simulink model "Quaternions_Method_merge_main"  (R2021b)
settings: Solver=VariableStepAuto  StartTime=0.0  StopTime=Time  FixedStep=1e-1  RelTol=1e-13  AbsTol=1e-8
values from neighbouring files (symbols this model uses):
  a = 8.6251e06    (= 8625100)    [main_code.m]
  A_BN_0 = eye(3)    [main_code.m]
  A_rw = [1 0 0 1/sqrt(3);         0 1 0 1/sqrt(3) ... (first row only)    [main_code.m]
  A_rw_star = [5/6 -1/6 -1/6;              -1/6  5/6 -1/6 ... (first row only)    [main_code.m]
  c = 2.99792*10^8    (= 299792000)    [main_code.m]
  e = 0.1195    [main_code.m]
  i = 0.3815    [main_code.m]
  MB = [1; 0.3; 0.3; 0.3]    [main_code.m]
  mr = 1.2*1e-4    (= 0.00012)    [main_code.m]
  omega_0 = [w_0x; w_0y; w_0z]    [main_code.m]
  sig_b = sig_b^2    [main_code.m]
  sig_n = 0.15*pi/180/3600/sqrt(t_sample)    [main_code.m]
  SP = [3; 0.3; 1; 0.1]    [main_code.m]
  T = 2*pi / n    [main_code.m]
  t_sample = 1    [main_code.m]
undefined symbols (not defined in the file or in its folder): f_mag, H_0, magnitude, muP, p_acc, RD, RS_MB, RS_SP, theta0, w_E
libraries: matrix_library x14, vrlib x8, simulink x2, simulink_extras x1
(part 5 of 5)

== matlab function Quaternions_Method_merge_main/Attitude determination/MATLAB Function ==
  data: K input; V output; D output
function [V, D] = fcn(K)
[V,D] = eig(K);
end

== matlab function Quaternions_Method_merge_main/Enviroment/Magnetic torque /Magnetic torque in body frame/MATLAB Function ==
  data: R input; r_LVLH input; t input; teta input; B_N output
function B_N = fcn(R, r_LVLH, t, teta)

%% First thing is to define the vector containing all the polynimials up to the 4th order
P1 = 1;
P2 = teta;
P3 = ((3*teta^2)-1)/2;
P4 = ((5*teta^3)-(3*teta))/2;

% Computing the derivatives of the P polynomials
P1_der = 0;
P2_der = 1;
P3_der = 3*teta;
P4_der = ((15*teta^2)-3)/2;

r = norm(r_LVLH);
% Defining the order of the approximation k 
k = 4;

% Defining the matrices containing the coefficients needed to make the
% approximation model IGRF2000 (following the tables on the slide number 5 of the
% pack of slides number 8)
g = 1e9*[-29615 -1728 0 0 0; ...
                      -2267 3072 1672 0 0; ...
                     1341 -2290 1253 715 0; ...
                     935 787 251 -405 110]; %[T]
h = 1e9*[0 5186 0 0 0; ...
                     0 -2478 -458 0 0; ...
                     0 -227 296 -492 0; ...
                     0 272 -232 119 -304]; %[T]

% Computing the right ascension alpha, the declination delta, the longitude lon and the co-latitude phi
delta = asin(r_LVLH(3)/r); %[rad]
if(r_LVLH(2)/r > 0)
    alpha = acos((r_LVLH(1)/r)/cos(delta)); %[rad]
else 
    alpha = 2*pi -  acos((r_LVLH(1)/r)/cos(delta)); %[rad]
end
lat = -delta; %[rad]
phi = pi - lat; %[rad]
om_E = deg2rad(15.04)/3600; 
Gren_lon = om_E*t;
lon = (alpha - Gren_lon);

% Computing the for cicle to obtain components of B in r, th, phi RF
b_r = [];
b_th = [];
b_phi = [];
P_mat = [];
P_matder = [];
b1 = [];
b2 = [];
b3 = [];

syms v;
for n = 1:k
    P5 = (v^2-1)^n;
    Df1 = diff(P5,v,n);
    P_poly = 1/((2^n)*factorial(n))*Df1(teta);
    for m = 1:(n+1)
%         P_mat = (2*factorial(n-m))/factorial(n+m)*[P1, P1, P1, P1; P2, P2, P2, P2; P3, P3, P3, P3; P4, P4, P4, P4];
%         P_matder = ((2*factorial(n-m))/factorial(n+m))*[P1_der, P1_der, P1_der, P1_der; P2_der, P2_der, P2_der, P2_der; P3_der, P3_der, P3_der, P3_der; P4_der, P4_der, P4_der, P4_der];
%         b_r = (R/r)^n+2*(n+1)*((g(n, m)*cos(m*phi)+h(n,m)*sin(m*phi))*P_mat(n,m));
%         b_th = -(R/r)^(n+2)*((g(n, m)*cos(m*phi)+h(n,m)*sin(m*phi))*P_matder(n,m));
%         b_phi = -1/sin(teta)*((R/r)^(n+2))*((-g(n,m)*sin(m*phi) + h(n,m)*cos(m*phi))*P_mat(n,m));
          Df2 = diff(P_poly,v,m);
          Df3 = diff(P6,v, m);
          P6 = sqrt(((2*factorial(n-m))/factorial(n+m)))*((1-v^2)^1/(2*m))*Df2(teta);
          b_r = (R/r)^n+2*(n+1)*(g(n, m)*cos(m*phi)+h(n,m)*sin(m*phi))*sqrt(((2*factorial(n-m))/factorial(n+m)))*((1-v^2)^1/(2*m))*Df2(teta);
          b_th = -(R/r)^(n+2)*((g(n, m)*cos(m*phi)+h(n,m)*sin(m*phi))*P_matder(n,m))*Df3(teta);
          b_phi = -1/sin(teta)*((R/r)^(n+2))*((-g(n,m)*sin(m*phi) + h(n,m)*cos(m*phi))*P_mat(n,m))*sqrt(((2*factorial(n-m))/factorial(n+m)))*((1-v^2)^1/(2*m))*Df2(teta);

        % Computing the magnetic torque in the inertial frame 
        b1 = (b_r*cos(delta)+b_th*sin(delta))*cos(alpha)-b_phi*sin(alpha);
        b2 = (b_r*cos(delta)+b_th*sin(delta))*sin(alpha)+b_phi*cos(alpha);
        b3 = b_r*sin(delta)-b_th*cos(delta);
    end
end
B_N = [b1; b2; b3];


end

== matlab function Quaternions_Method_merge_main/Enviroment/Magnetic torque /Magnetic torque in body frame/MATLAB Function1 ==
  data: r input; Br output; theta input; phi input; days input; Bt output; Bp output
function [Br,Bt,Bp] = magnet(r,theta,phi,days)
% Inputs
% r Geocentric radius
% theta Latitude measured in degrees positive from equator
% phi Longitude measured in degrees positive east from Greenwich
% days Decimal days since January 1, 2000
%
% Outputs - magnetic field strength in local tangential coordinates
% Br B in radial direction
% Bt B in theta direction
% Bp B in phi direction
% Checks to see if located at either pole to avoid singularities
if (theta>-0.00000001 & theta<0.00000001)
theta=0.00000001;
elseif(theta<180.00000001 & theta>179.99999999)
theta=179.99999999;
end
% The angles must be converted from degrees into radians
theta=(90-theta)*pi/180;
phi = phi*pi/180;
a=6371.2; % Reference radius used in IGRF
% This section of the code simply reads in the g and h Schmidt
% quasi-normalized coefficients
[gn, gm, gvali, gsvi] = textread(’igrfSg.txt’,’%f %f %f %f’);
[hn, hm, hvali, hsvi] = textread(’igrfSh.txt’,’%f %f %f %f’);
N=max(gn);
g=zeros(N,N+1);
h=zeros(N,N+1);
for x=1:length(gn)
g(gn(x),gm(x)+1) = gvali(x) + gsvi(x)*days/365;
h(hn(x),hm(x)+1) = hvali(x) + hsvi(x)*days/365;
end
% Initialize each of the variables
% Br B in the radial driection
% Bt B in the theta direction
12
% Bp B in the phi direction
% P The associated Legendre polynomial evaluated at cos(theta)
% The nomenclature for the recursive values generally follows
% the form P10 = P(n-1,m-0)
% dP The partial derivative of P with respect to theta
Br=0; Bt=0; Bp=0;
P11=1; P10=P11;
dP11=0; dP10=dP11;
for m=0:N
for n=1:N
if m<=n
% Calculate Legendre polynomials and derivatives recursively
if n==m
P2 = sin(theta)*P11;
dP2 = sin(theta)*dP11 + cos(theta)*P11;
P11=P2; P10=P11; P20=0;
dP11=dP2; dP10=dP11; dP20=0;
elseif n==1
P2 = cos(theta)*P10;
dP2 = cos(theta)*dP10 - sin(theta)*P10;
P20=P10; P10=P2;
dP20=dP10; dP10=dP2;
else
K = ((n-1)^2-m^2)/((2*n-1)*(2*n-3));
P2 = cos(theta)*P10 - K*P20;
dP2 = cos(theta)*dP10 - sin(theta)*P10 - K*dP20;
P20=P10; P10=P2;
dP20=dP10; dP10=dP2;
end
% Calculate Br, Bt, and Bp
Br = Br + (a/r)^(n+2)*(n+1)*...
((g(n,m+1)*cos(m*phi) + h(n,m+1)*sin(m*phi))*P2);
Bt = Bt + (a/r)^(n+2)*...
((g(n,m+1)*cos(m*phi) + h(n,m+1)*sin(m*phi))*dP2);
Bp = Bp + (a/r)^(n+2)*...
(m*(-g(n,m+1)*sin(m*phi) + h(n,m+1)*cos(m*phi))* P2);
end
end
end
[Br,Bt,Bp] = [Br;-Bt;-Bp/sin(theta)];
